simulink model "PID"  (R2023a)
settings: Solver=VariableStepAuto  StartTime=0.0  StopTime=1000  RelTol=1e-3
PreLoadFcn:
  | eta = Simulink.Signal;
  | eta.CoderInfo.StorageClass = 'ExportedGlobal';
  | eta.InitialValue = '[0 0 0 0 0 0]';
  | V = Simulink.Signal;
  | V.CoderInfo.StorageClass = 'ExportedGlobal';
  | V.InitialValue = '[0 0 0 0 0 0]';
model workspace: external: MATLAB File /home/ponbapanda/study_material/ee4901/6DOF-UUV/src/OdeRexRov.m (data not in the file)
values from neighbouring files (symbols this model uses):
  Minv = inv(M)    [OdeRexRov.m]
undefined symbols (not defined in the file or in its folder): DiscIntNeverNeededParam
libraries: slpidlib x6, simulink x1
settings Model: Creator=ponbapanda  LastModifiedBy=ponbapanda

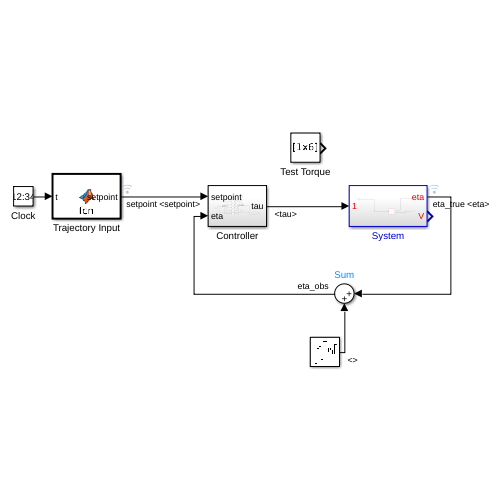
[thumbnail: Simulink's stored preview of the top-level diagram]
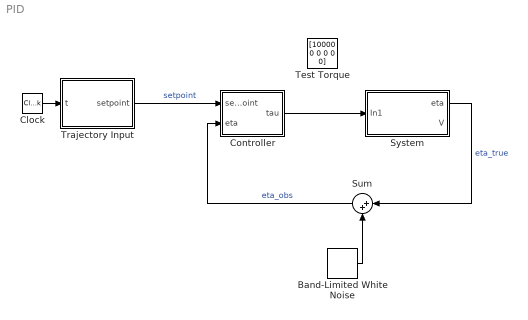
== system PID ==
  Band-Limited White Noise : simulink/Sources/Band-Limited White Noise  Cov=[0.1 0.1 0.1 0.05 0.05 0.05]  Ts=0.05  seed=[23341]
  Clock : DigitalClock  SampleTime=0.05
  Controller : Subsystem
  Sum : Sum  Inputs=|++
  System : Subsystem
  Test Torque : Constant  Value=[10000 0 0 0 0 0]
  Trajectory Input : MATLAB Function  TreatAsAtomicUnit=on
  wires:
  Clock/1 -> Trajectory Input/1(t)
  Trajectory Input/1(setpoint) -> Controller/1(setpoint)  "setpoint"
  System/1(eta) -> Sum/1  "eta_true"
  Controller/1(tau) -> System/1(In1)
  Band-Limited White Noise/1 -> Sum/2
  Sum/1 -> Controller/2(eta)  "eta_obs"

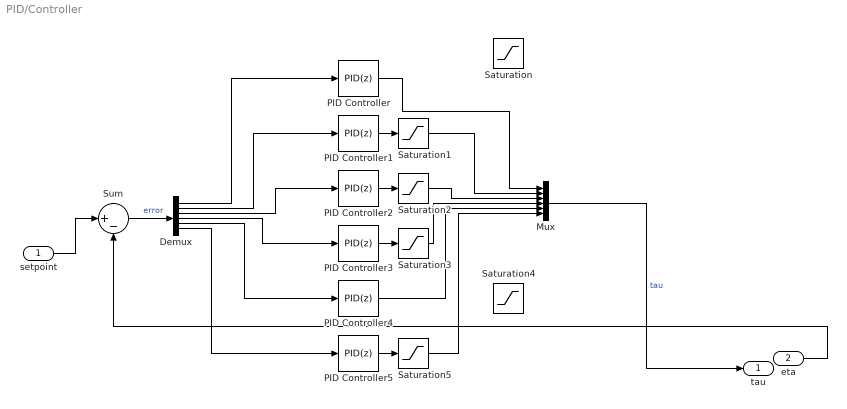
== system PID/Controller ==
  setpoint : Inport
  eta : Inport  Port=2
  Demux : Demux  Outputs=6
  Mux : Mux  Inputs=6
  PID Controller : slpidlib/PID Controller  Controller=PID  Form=Parallel  TimeDomain=Discrete-time  UseExternalTs=off  SampleTime=0.0500000000000000028  IntegratorMethod=Forward Euler  FilterMethod=Forward Euler  ControllerParametersSource=internal  P=500.000000000000000  I=10.000000000000000  UseKiTs=off  D=503.391827453152189  N=19.865241060018288  UseFilter=on  TunerSelectOption=Transfer Function Based (PID Tuner App)  InitialConditionSource=internal  InitialConditionForIntegrator=0  InitialConditionForFilter=0  DifferentiatorICPrevScaledInput=0  ExternalReset=none  TrackingMode=off  Kt=1  LimitOutput=off  SatLimitsSource=internal  UpperSaturationLimit=inf  LowerSaturationLimit=-inf  LinearizeAsGain=on  AntiWindupMode=none  Kb=1  LimitIntegrator=off  UpperIntegratorSaturationLimit=inf  LowerIntegratorSaturationLimit=-inf  POutMin=[]  POutMax=[]  IOutMin=[]  IOutMax=[]  DOutMin=[]  DOutMax=[]  NOutMin=[]  NOutMax=[]  SumOutMin=[]  SumOutMax=[]  SaturationOutMin=[]  SaturationOutMax=[]  PParamMin=[]  PParamMax=[]  IParamMin=[]  IParamMax=[]  DParamMin=[]  DParamMax=[]  NParamMin=[]  NParamMax=[]  KbParamMin=[]  KbParamMax=[]  KtParamMin=[]  KtParamMax=[]  KbOutMin=[]  KbOutMax=[]  KtOutMin=[]  KtOutMax=[]  IntegratorOutMin=[]  IntegratorOutMax=[]  FilterOutMin=[]  FilterOutMax=[]  SumI1OutMin=[]  SumI1OutMax=[]  SumI2OutMin=[]  SumI2OutMax=[]  SumI3OutMin=[]  SumI3OutMax=[]  SumI4OutMin=[]  SumI4OutMax=[]  SumDOutMin=[]  SumDOutMax=[]  DifferentiatorOutMin=[]  DifferentiatorOutMax=[]  FilterDiffOutCoefMin=[]  FilterDiffOutCoefMax=[]  ReciprocalOutMin=[]  ReciprocalOutMax=[]  SumDenOutMin=[]  SumDenOutMax=[]  SumNumOutMin=[]  SumNumOutMax=[]  DivideOutMin=[]  DivideOutMax=[]  UdiffTsProdOutMin=[]  UdiffTsProdOutMax=[]  NTsProdOutMin=[]  NTsProdOutMax=[]  UintegralTsProdOutMin=[]  UintegralTsProdOutMax=[]  UngainTsProdOutMin=[]  UngainTsProdOutMax=[]  ClampingZeroOutDataTypeStr=Inherit: Inherit via back propagation  ClampingZeroOutMin=[]  ClampingZeroOutMax=[]  FilterDenConstantOutDataTypeStr=Inherit: Inherit via back propagation  FilterDenConstantOutMin=[]  FilterDenConstantOutMax=[]  PCopyOutDataTypeStr=Inherit: Inherit via back propagation  PCopyOutMin=[]  PCopyOutMax=[]  NCopyOutDataTypeStr=Inherit: Inherit via back propagation  NCopyOutMin=[]  NCopyOutMax=[]  IntegratorContinuousStateAttributes=''  IntegratorStateMustResolveToSignalObject=off  IntegratorRTWStateStorageClass=Auto  FilterContinuousStateAttributes=''  FilterStateMustResolveToSignalObject=off  FilterRTWStateStorageClass=Auto  ParallelPVariant=InternalParameters  IdealPVariant=Disabled  IVariant=InternalParameters  DVariant=InternalParameters  IntegratorVariant=Discrete  SatVariant=Disabled  AWVariant=Passthrough  PCopyVariant=Disabled  TRVariant=Disabled  FdbkBlocksVariant=Forward  IdealPFdbkVariant=Disabled  SatFdbkVariant=Disabled  DerivativeFilterVariant=ForwardEulerFilter  NVariant=InternalParameters  NCopyVariant=Disabled  FilterICVariant=InternalICsFilter  IntegratorICVariant=InternalICs  ExternalResetVariant=Disabled  TRSumVariant=Passthrough  SumFdbkVariant=Disabled  SumVariant=Sum_PID  TsampFilterVariant=InternalTs  TsampNgainVariant=Passthrough  TsampIntegralVariant=Disabled_SignalSpec  ExternalSaturationOutDataTypeStr=Inherit: Same as second input
  PID Controller1 : slpidlib/PID Controller  Controller=PID  Form=Parallel  TimeDomain=Discrete-time  UseExternalTs=off  SampleTime=0.0500000000000000028  IntegratorMethod=Forward Euler  FilterMethod=Forward Euler  ControllerParametersSource=internal  P=500.000000000000000  I=10.000000000000000  UseKiTs=off  D=503.391827453152189  N=19.865241060018288  UseFilter=on  TunerSelectOption=Transfer Function Based (PID Tuner App)  InitialConditionSource=internal  InitialConditionForIntegrator=0  InitialConditionForFilter=0  DifferentiatorICPrevScaledInput=0  ExternalReset=none  TrackingMode=off  Kt=1  LimitOutput=off  SatLimitsSource=internal  UpperSaturationLimit=inf  LowerSaturationLimit=-inf  LinearizeAsGain=on  AntiWindupMode=none  Kb=1  LimitIntegrator=off  UpperIntegratorSaturationLimit=inf  LowerIntegratorSaturationLimit=-inf  POutMin=[]  POutMax=[]  IOutMin=[]  IOutMax=[]  DOutMin=[]  DOutMax=[]  NOutMin=[]  NOutMax=[]  SumOutMin=[]  SumOutMax=[]  SaturationOutMin=[]  SaturationOutMax=[]  PParamMin=[]  PParamMax=[]  IParamMin=[]  IParamMax=[]  DParamMin=[]  DParamMax=[]  NParamMin=[]  NParamMax=[]  KbParamMin=[]  KbParamMax=[]  KtParamMin=[]  KtParamMax=[]  KbOutMin=[]  KbOutMax=[]  KtOutMin=[]  KtOutMax=[]  IntegratorOutMin=[]  IntegratorOutMax=[]  FilterOutMin=[]  FilterOutMax=[]  SumI1OutMin=[]  SumI1OutMax=[]  SumI2OutMin=[]  SumI2OutMax=[]  SumI3OutMin=[]  SumI3OutMax=[]  SumI4OutMin=[]  SumI4OutMax=[]  SumDOutMin=[]  SumDOutMax=[]  DifferentiatorOutMin=[]  DifferentiatorOutMax=[]  FilterDiffOutCoefMin=[]  FilterDiffOutCoefMax=[]  ReciprocalOutMin=[]  ReciprocalOutMax=[]  SumDenOutMin=[]  SumDenOutMax=[]  SumNumOutMin=[]  SumNumOutMax=[]  DivideOutMin=[]  DivideOutMax=[]  UdiffTsProdOutMin=[]  UdiffTsProdOutMax=[]  NTsProdOutMin=[]  NTsProdOutMax=[]  UintegralTsProdOutMin=[]  UintegralTsProdOutMax=[]  UngainTsProdOutMin=[]  UngainTsProdOutMax=[]  ClampingZeroOutDataTypeStr=Inherit: Inherit via back propagation  ClampingZeroOutMin=[]  ClampingZeroOutMax=[]  FilterDenConstantOutDataTypeStr=Inherit: Inherit via back propagation  FilterDenConstantOutMin=[]  FilterDenConstantOutMax=[]  PCopyOutDataTypeStr=Inherit: Inherit via back propagation  PCopyOutMin=[]  PCopyOutMax=[]  NCopyOutDataTypeStr=Inherit: Inherit via back propagation  NCopyOutMin=[]  NCopyOutMax=[]  IntegratorContinuousStateAttributes=''  IntegratorStateMustResolveToSignalObject=off  IntegratorRTWStateStorageClass=Auto  FilterContinuousStateAttributes=''  FilterStateMustResolveToSignalObject=off  FilterRTWStateStorageClass=Auto  ParallelPVariant=InternalParameters  IdealPVariant=Disabled  IVariant=InternalParameters  DVariant=InternalParameters  IntegratorVariant=Discrete  SatVariant=Disabled  AWVariant=Passthrough  PCopyVariant=Disabled  TRVariant=Disabled  FdbkBlocksVariant=Forward  IdealPFdbkVariant=Disabled  SatFdbkVariant=Disabled  DerivativeFilterVariant=ForwardEulerFilter  NVariant=InternalParameters  NCopyVariant=Disabled  FilterICVariant=InternalICsFilter  IntegratorICVariant=InternalICs  ExternalResetVariant=Disabled  TRSumVariant=Passthrough  SumFdbkVariant=Disabled  SumVariant=Sum_PID  TsampFilterVariant=InternalTs  TsampNgainVariant=Passthrough  TsampIntegralVariant=Disabled_SignalSpec  ExternalSaturationOutDataTypeStr=Inherit: Same as second input
  PID Controller2 : slpidlib/PID Controller  Controller=PID  Form=Parallel  TimeDomain=Discrete-time  UseExternalTs=off  SampleTime=0.0500000000000000028  IntegratorMethod=Forward Euler  FilterMethod=Forward Euler  ControllerParametersSource=internal  P=500.000000000000000  I=0.000000000000000  UseKiTs=off  D=503.391827453152189  N=19.865241060018288  UseFilter=on  TunerSelectOption=Transfer Function Based (PID Tuner App)  InitialConditionSource=internal  InitialConditionForIntegrator=0  InitialConditionForFilter=0  DifferentiatorICPrevScaledInput=0  ExternalReset=none  TrackingMode=off  Kt=1  LimitOutput=off  SatLimitsSource=internal  UpperSaturationLimit=inf  LowerSaturationLimit=-inf  LinearizeAsGain=on  AntiWindupMode=none  Kb=1  LimitIntegrator=off  UpperIntegratorSaturationLimit=inf  LowerIntegratorSaturationLimit=-inf  POutMin=[]  POutMax=[]  IOutMin=[]  IOutMax=[]  DOutMin=[]  DOutMax=[]  NOutMin=[]  NOutMax=[]  SumOutMin=[]  SumOutMax=[]  SaturationOutMin=[]  SaturationOutMax=[]  PParamMin=[]  PParamMax=[]  IParamMin=[]  IParamMax=[]  DParamMin=[]  DParamMax=[]  NParamMin=[]  NParamMax=[]  KbParamMin=[]  KbParamMax=[]  KtParamMin=[]  KtParamMax=[]  KbOutMin=[]  KbOutMax=[]  KtOutMin=[]  KtOutMax=[]  IntegratorOutMin=[]  IntegratorOutMax=[]  FilterOutMin=[]  FilterOutMax=[]  SumI1OutMin=[]  SumI1OutMax=[]  SumI2OutMin=[]  SumI2OutMax=[]  SumI3OutMin=[]  SumI3OutMax=[]  SumI4OutMin=[]  SumI4OutMax=[]  SumDOutMin=[]  SumDOutMax=[]  DifferentiatorOutMin=[]  DifferentiatorOutMax=[]  FilterDiffOutCoefMin=[]  FilterDiffOutCoefMax=[]  ReciprocalOutMin=[]  ReciprocalOutMax=[]  SumDenOutMin=[]  SumDenOutMax=[]  SumNumOutMin=[]  SumNumOutMax=[]  DivideOutMin=[]  DivideOutMax=[]  UdiffTsProdOutMin=[]  UdiffTsProdOutMax=[]  NTsProdOutMin=[]  NTsProdOutMax=[]  UintegralTsProdOutMin=[]  UintegralTsProdOutMax=[]  UngainTsProdOutMin=[]  UngainTsProdOutMax=[]  ClampingZeroOutDataTypeStr=Inherit: Inherit via back propagation  ClampingZeroOutMin=[]  ClampingZeroOutMax=[]  FilterDenConstantOutDataTypeStr=Inherit: Inherit via back propagation  FilterDenConstantOutMin=[]  FilterDenConstantOutMax=[]  PCopyOutDataTypeStr=Inherit: Inherit via back propagation  PCopyOutMin=[]  PCopyOutMax=[]  NCopyOutDataTypeStr=Inherit: Inherit via back propagation  NCopyOutMin=[]  NCopyOutMax=[]  IntegratorContinuousStateAttributes=''  IntegratorStateMustResolveToSignalObject=off  IntegratorRTWStateStorageClass=Auto  FilterContinuousStateAttributes=''  FilterStateMustResolveToSignalObject=off  FilterRTWStateStorageClass=Auto  ParallelPVariant=InternalParameters  IdealPVariant=Disabled  IVariant=InternalParameters  DVariant=InternalParameters  IntegratorVariant=Discrete  SatVariant=Disabled  AWVariant=Passthrough  PCopyVariant=Disabled  TRVariant=Disabled  FdbkBlocksVariant=Forward  IdealPFdbkVariant=Disabled  SatFdbkVariant=Disabled  DerivativeFilterVariant=ForwardEulerFilter  NVariant=InternalParameters  NCopyVariant=Disabled  FilterICVariant=InternalICsFilter  IntegratorICVariant=InternalICs  ExternalResetVariant=Disabled  TRSumVariant=Passthrough  SumFdbkVariant=Disabled  SumVariant=Sum_PID  TsampFilterVariant=InternalTs  TsampNgainVariant=Passthrough  TsampIntegralVariant=Disabled_SignalSpec  ExternalSaturationOutDataTypeStr=Inherit: Same as second input
  PID Controller3 : slpidlib/PID Controller  Controller=PID  Form=Parallel  TimeDomain=Discrete-time  UseExternalTs=off  SampleTime=0.0500000000000000028  IntegratorMethod=Forward Euler  FilterMethod=Forward Euler  ControllerParametersSource=internal  P=5000.000000000000000  I=500.000000000000000  UseKiTs=off  D=503.391827453152189  N=19.865241060018288  UseFilter=on  TunerSelectOption=Transfer Function Based (PID Tuner App)  InitialConditionSource=internal  InitialConditionForIntegrator=0  InitialConditionForFilter=0  DifferentiatorICPrevScaledInput=0  ExternalReset=none  TrackingMode=off  Kt=1  LimitOutput=off  SatLimitsSource=internal  UpperSaturationLimit=inf  LowerSaturationLimit=-inf  LinearizeAsGain=on  AntiWindupMode=none  Kb=1  LimitIntegrator=off  UpperIntegratorSaturationLimit=inf  LowerIntegratorSaturationLimit=-inf  POutMin=[]  POutMax=[]  IOutMin=[]  IOutMax=[]  DOutMin=[]  DOutMax=[]  NOutMin=[]  NOutMax=[]  SumOutMin=[]  SumOutMax=[]  SaturationOutMin=[]  SaturationOutMax=[]  PParamMin=[]  PParamMax=[]  IParamMin=[]  IParamMax=[]  DParamMin=[]  DParamMax=[]  NParamMin=[]  NParamMax=[]  KbParamMin=[]  KbParamMax=[]  KtParamMin=[]  KtParamMax=[]  KbOutMin=[]  KbOutMax=[]  KtOutMin=[]  KtOutMax=[]  IntegratorOutMin=[]  IntegratorOutMax=[]  FilterOutMin=[]  FilterOutMax=[]  SumI1OutMin=[]  SumI1OutMax=[]  SumI2OutMin=[]  SumI2OutMax=[]  SumI3OutMin=[]  SumI3OutMax=[]  SumI4OutMin=[]  SumI4OutMax=[]  SumDOutMin=[]  SumDOutMax=[]  DifferentiatorOutMin=[]  DifferentiatorOutMax=[]  FilterDiffOutCoefMin=[]  FilterDiffOutCoefMax=[]  ReciprocalOutMin=[]  ReciprocalOutMax=[]  SumDenOutMin=[]  SumDenOutMax=[]  SumNumOutMin=[]  SumNumOutMax=[]  DivideOutMin=[]  DivideOutMax=[]  UdiffTsProdOutMin=[]  UdiffTsProdOutMax=[]  NTsProdOutMin=[]  NTsProdOutMax=[]  UintegralTsProdOutMin=[]  UintegralTsProdOutMax=[]  UngainTsProdOutMin=[]  UngainTsProdOutMax=[]  ClampingZeroOutDataTypeStr=Inherit: Inherit via back propagation  ClampingZeroOutMin=[]  ClampingZeroOutMax=[]  FilterDenConstantOutDataTypeStr=Inherit: Inherit via back propagation  FilterDenConstantOutMin=[]  FilterDenConstantOutMax=[]  PCopyOutDataTypeStr=Inherit: Inherit via back propagation  PCopyOutMin=[]  PCopyOutMax=[]  NCopyOutDataTypeStr=Inherit: Inherit via back propagation  NCopyOutMin=[]  NCopyOutMax=[]  IntegratorContinuousStateAttributes=''  IntegratorStateMustResolveToSignalObject=off  IntegratorRTWStateStorageClass=Auto  FilterContinuousStateAttributes=''  FilterStateMustResolveToSignalObject=off  FilterRTWStateStorageClass=Auto  ParallelPVariant=InternalParameters  IdealPVariant=Disabled  IVariant=InternalParameters  DVariant=InternalParameters  IntegratorVariant=Discrete  SatVariant=Disabled  AWVariant=Passthrough  PCopyVariant=Disabled  TRVariant=Disabled  FdbkBlocksVariant=Forward  IdealPFdbkVariant=Disabled  SatFdbkVariant=Disabled  DerivativeFilterVariant=ForwardEulerFilter  NVariant=InternalParameters  NCopyVariant=Disabled  FilterICVariant=InternalICsFilter  IntegratorICVariant=InternalICs  ExternalResetVariant=Disabled  TRSumVariant=Passthrough  SumFdbkVariant=Disabled  SumVariant=Sum_PID  TsampFilterVariant=InternalTs  TsampNgainVariant=Passthrough  TsampIntegralVariant=Disabled_SignalSpec  ExternalSaturationOutDataTypeStr=Inherit: Same as second input
  PID Controller4 : slpidlib/PID Controller  Controller=PID  Form=Parallel  TimeDomain=Discrete-time  UseExternalTs=off  SampleTime=0.0500000000000000028  IntegratorMethod=Forward Euler  FilterMethod=Forward Euler  ControllerParametersSource=internal  P=5000.000000000000000  I=500.000000000000000  UseKiTs=off  D=503.391827453152189  N=19.865241060018288  UseFilter=on  TunerSelectOption=Transfer Function Based (PID Tuner App)  InitialConditionSource=internal  InitialConditionForIntegrator=0  InitialConditionForFilter=0  DifferentiatorICPrevScaledInput=0  ExternalReset=none  TrackingMode=off  Kt=1  LimitOutput=off  SatLimitsSource=internal  UpperSaturationLimit=inf  LowerSaturationLimit=-inf  LinearizeAsGain=on  AntiWindupMode=none  Kb=1  LimitIntegrator=off  UpperIntegratorSaturationLimit=inf  LowerIntegratorSaturationLimit=-inf  POutMin=[]  POutMax=[]  IOutMin=[]  IOutMax=[]  DOutMin=[]  DOutMax=[]  NOutMin=[]  NOutMax=[]  SumOutMin=[]  SumOutMax=[]  SaturationOutMin=[]  SaturationOutMax=[]  PParamMin=[]  PParamMax=[]  IParamMin=[]  IParamMax=[]  DParamMin=[]  DParamMax=[]  NParamMin=[]  NParamMax=[]  KbParamMin=[]  KbParamMax=[]  KtParamMin=[]  KtParamMax=[]  KbOutMin=[]  KbOutMax=[]  KtOutMin=[]  KtOutMax=[]  IntegratorOutMin=[]  IntegratorOutMax=[]  FilterOutMin=[]  FilterOutMax=[]  SumI1OutMin=[]  SumI1OutMax=[]  SumI2OutMin=[]  SumI2OutMax=[]  SumI3OutMin=[]  SumI3OutMax=[]  SumI4OutMin=[]  SumI4OutMax=[]  SumDOutMin=[]  SumDOutMax=[]  DifferentiatorOutMin=[]  DifferentiatorOutMax=[]  FilterDiffOutCoefMin=[]  FilterDiffOutCoefMax=[]  ReciprocalOutMin=[]  ReciprocalOutMax=[]  SumDenOutMin=[]  SumDenOutMax=[]  SumNumOutMin=[]  SumNumOutMax=[]  DivideOutMin=[]  DivideOutMax=[]  UdiffTsProdOutMin=[]  UdiffTsProdOutMax=[]  NTsProdOutMin=[]  NTsProdOutMax=[]  UintegralTsProdOutMin=[]  UintegralTsProdOutMax=[]  UngainTsProdOutMin=[]  UngainTsProdOutMax=[]  ClampingZeroOutDataTypeStr=Inherit: Inherit via back propagation  ClampingZeroOutMin=[]  ClampingZeroOutMax=[]  FilterDenConstantOutDataTypeStr=Inherit: Inherit via back propagation  FilterDenConstantOutMin=[]  FilterDenConstantOutMax=[]  PCopyOutDataTypeStr=Inherit: Inherit via back propagation  PCopyOutMin=[]  PCopyOutMax=[]  NCopyOutDataTypeStr=Inherit: Inherit via back propagation  NCopyOutMin=[]  NCopyOutMax=[]  IntegratorContinuousStateAttributes=''  IntegratorStateMustResolveToSignalObject=off  IntegratorRTWStateStorageClass=Auto  FilterContinuousStateAttributes=''  FilterStateMustResolveToSignalObject=off  FilterRTWStateStorageClass=Auto  ParallelPVariant=InternalParameters  IdealPVariant=Disabled  IVariant=InternalParameters  DVariant=InternalParameters  IntegratorVariant=Discrete  SatVariant=Disabled  AWVariant=Passthrough  PCopyVariant=Disabled  TRVariant=Disabled  FdbkBlocksVariant=Forward  IdealPFdbkVariant=Disabled  SatFdbkVariant=Disabled  DerivativeFilterVariant=ForwardEulerFilter  NVariant=InternalParameters  NCopyVariant=Disabled  FilterICVariant=InternalICsFilter  IntegratorICVariant=InternalICs  ExternalResetVariant=Disabled  TRSumVariant=Passthrough  SumFdbkVariant=Disabled  SumVariant=Sum_PID  TsampFilterVariant=InternalTs  TsampNgainVariant=Passthrough  TsampIntegralVariant=Disabled_SignalSpec  ExternalSaturationOutDataTypeStr=Inherit: Same as second input
  PID Controller5 : slpidlib/PID Controller  Controller=PID  Form=Parallel  TimeDomain=Discrete-time  UseExternalTs=off  SampleTime=0.0500000000000000028  IntegratorMethod=Forward Euler  FilterMethod=Forward Euler  ControllerParametersSource=internal  P=5000.000000000000000  I=500.000000000000000  UseKiTs=off  D=503.391827453152189  N=19.865241060018288  UseFilter=on  TunerSelectOption=Transfer Function Based (PID Tuner App)  InitialConditionSource=internal  InitialConditionForIntegrator=0  InitialConditionForFilter=0  DifferentiatorICPrevScaledInput=0  ExternalReset=none  TrackingMode=off  Kt=1  LimitOutput=off  SatLimitsSource=internal  UpperSaturationLimit=inf  LowerSaturationLimit=-inf  LinearizeAsGain=on  AntiWindupMode=none  Kb=1  LimitIntegrator=off  UpperIntegratorSaturationLimit=inf  LowerIntegratorSaturationLimit=-inf  POutMin=[]  POutMax=[]  IOutMin=[]  IOutMax=[]  DOutMin=[]  DOutMax=[]  NOutMin=[]  NOutMax=[]  SumOutMin=[]  SumOutMax=[]  SaturationOutMin=[]  SaturationOutMax=[]  PParamMin=[]  PParamMax=[]  IParamMin=[]  IParamMax=[]  DParamMin=[]  DParamMax=[]  NParamMin=[]  NParamMax=[]  KbParamMin=[]  KbParamMax=[]  KtParamMin=[]  KtParamMax=[]  KbOutMin=[]  KbOutMax=[]  KtOutMin=[]  KtOutMax=[]  IntegratorOutMin=[]  IntegratorOutMax=[]  FilterOutMin=[]  FilterOutMax=[]  SumI1OutMin=[]  SumI1OutMax=[]  SumI2OutMin=[]  SumI2OutMax=[]  SumI3OutMin=[]  SumI3OutMax=[]  SumI4OutMin=[]  SumI4OutMax=[]  SumDOutMin=[]  SumDOutMax=[]  DifferentiatorOutMin=[]  DifferentiatorOutMax=[]  FilterDiffOutCoefMin=[]  FilterDiffOutCoefMax=[]  ReciprocalOutMin=[]  ReciprocalOutMax=[]  SumDenOutMin=[]  SumDenOutMax=[]  SumNumOutMin=[]  SumNumOutMax=[]  DivideOutMin=[]  DivideOutMax=[]  UdiffTsProdOutMin=[]  UdiffTsProdOutMax=[]  NTsProdOutMin=[]  NTsProdOutMax=[]  UintegralTsProdOutMin=[]  UintegralTsProdOutMax=[]  UngainTsProdOutMin=[]  UngainTsProdOutMax=[]  ClampingZeroOutDataTypeStr=Inherit: Inherit via back propagation  ClampingZeroOutMin=[]  ClampingZeroOutMax=[]  FilterDenConstantOutDataTypeStr=Inherit: Inherit via back propagation  FilterDenConstantOutMin=[]  FilterDenConstantOutMax=[]  PCopyOutDataTypeStr=Inherit: Inherit via back propagation  PCopyOutMin=[]  PCopyOutMax=[]  NCopyOutDataTypeStr=Inherit: Inherit via back propagation  NCopyOutMin=[]  NCopyOutMax=[]  IntegratorContinuousStateAttributes=''  IntegratorStateMustResolveToSignalObject=off  IntegratorRTWStateStorageClass=Auto  FilterContinuousStateAttributes=''  FilterStateMustResolveToSignalObject=off  FilterRTWStateStorageClass=Auto  ParallelPVariant=InternalParameters  IdealPVariant=Disabled  IVariant=InternalParameters  DVariant=InternalParameters  IntegratorVariant=Discrete  SatVariant=Disabled  AWVariant=Passthrough  PCopyVariant=Disabled  TRVariant=Disabled  FdbkBlocksVariant=Forward  IdealPFdbkVariant=Disabled  SatFdbkVariant=Disabled  DerivativeFilterVariant=ForwardEulerFilter  NVariant=InternalParameters  NCopyVariant=Disabled  FilterICVariant=InternalICsFilter  IntegratorICVariant=InternalICs  ExternalResetVariant=Disabled  TRSumVariant=Passthrough  SumFdbkVariant=Disabled  SumVariant=Sum_PID  TsampFilterVariant=InternalTs  TsampNgainVariant=Passthrough  TsampIntegralVariant=Disabled_SignalSpec  ExternalSaturationOutDataTypeStr=Inherit: Same as second input
  Saturation : Saturate  UpperLimit=8000  LowerLimit=-8000  LinearizeAsGain=off  ZeroCross=off
  Saturation1 : Saturate  UpperLimit=8000  LowerLimit=-8000  LinearizeAsGain=off  ZeroCross=off
  Saturation2 : Saturate  UpperLimit=8000  LowerLimit=-8000  LinearizeAsGain=off  ZeroCross=off
  Saturation3 : Saturate  UpperLimit=100000  LowerLimit=-100000  LinearizeAsGain=off  ZeroCross=off
  Saturation4 : Saturate  UpperLimit=100000  LowerLimit=-100000  LinearizeAsGain=off  ZeroCross=off
  Saturation5 : Saturate  UpperLimit=100000  LowerLimit=-100000  LinearizeAsGain=off  ZeroCross=off
  Sum : Sum  Inputs=|+-
  tau : Outport
  wires:
  PID Controller5/1 -> Saturation5/1
  setpoint/1 -> Sum/1
  PID Controller1/1 -> Saturation1/1
  Mux/1 -> tau/1  "tau"
  PID Controller4/1 -> Mux/5
  PID Controller/1 -> Mux/1
  Demux/5 -> PID Controller4/1
  eta/1 -> Sum/2
  PID Controller3/1 -> Saturation3/1
  Demux/2 -> PID Controller1/1
  Demux/4 -> PID Controller3/1
  Saturation2/1 -> Mux/3
  Demux/3 -> PID Controller2/1
  Demux/6 -> PID Controller5/1
  Saturation5/1 -> Mux/6
  Saturation3/1 -> Mux/4
  PID Controller2/1 -> Saturation2/1
  Sum/1 -> Demux/1  "error"
  Saturation1/1 -> Mux/2
  Demux/1 -> PID Controller/1

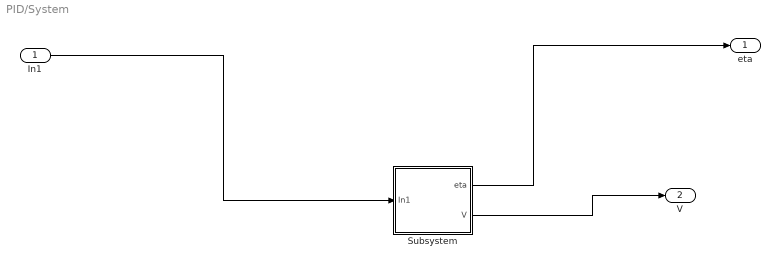
== system PID/System ==
  In1 : Inport
  Subsystem : Subsystem
  eta : Outport
  V : Outport  Port=2
  wires:
  In1/1 -> Subsystem/1(In1)
  Subsystem/1(eta) -> eta/1
  Subsystem/2(V) -> V/1

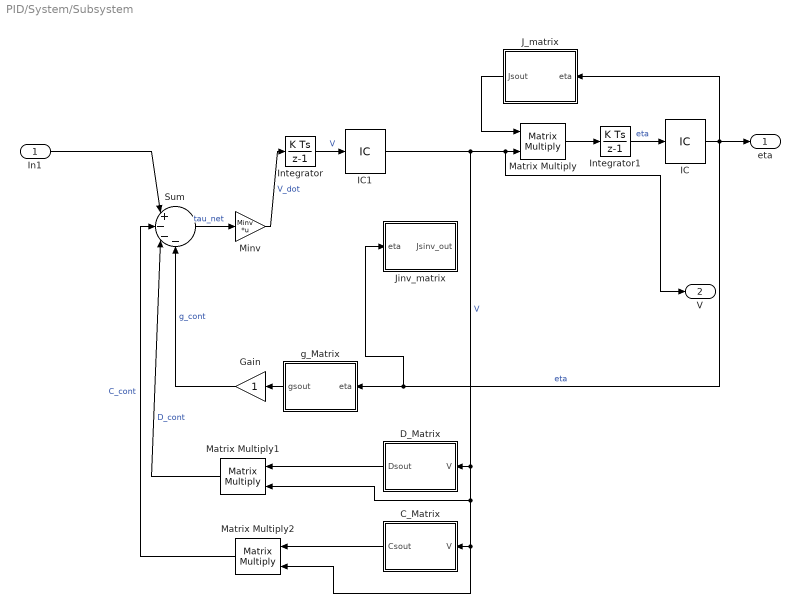
== system PID/System/Subsystem ==
  In1 : Inport
  C_Matrix : MATLAB Function  TreatAsAtomicUnit=on
  D_Matrix : MATLAB Function  TreatAsAtomicUnit=on
  Gain : Gain
  IC : InitialCondition  Value=[0 0 0 0 0 0]
  IC1 : InitialCondition  Value=[0 0 0 0 0 0]
  Integrator : DiscreteIntegrator  SampleTime=0.05  ICPrevOutput=DiscIntNeverNeededParam  ICPrevScaledInput=DiscIntNeverNeededParam  mask(DiscretizedDiscreteIntegrator){}
      mask init:
      | %zoh
  Integrator1 : DiscreteIntegrator  SampleTime=0.05  ICPrevOutput=DiscIntNeverNeededParam  ICPrevScaledInput=DiscIntNeverNeededParam  mask(DiscretizedDiscreteIntegrator){}
      mask init:
      | %zoh
  J_matrix : MATLAB Function  TreatAsAtomicUnit=on
  Jinv_matrix : MATLAB Function  TreatAsAtomicUnit=on
  Matrix Multiply : Product  Multiplication=Matrix(*)
  Matrix Multiply1 : Product  Multiplication=Matrix(*)
  Matrix Multiply2 : Product  Multiplication=Matrix(*)
  Minv : Gain  Gain=Minv  Multiplication=Matrix(K*u) (u vector)
  Sum : Sum  Inputs=|+---
  g_Matrix : MATLAB Function  TreatAsAtomicUnit=on
  eta : Outport
  V : Outport  Port=2
  wires:
  J_matrix/1(Jsout) -> Matrix Multiply/1
  Matrix Multiply1/1 -> Sum/3  "D_cont"
  Matrix Multiply2/1 -> Sum/2  "C_cont"
  D_Matrix/1(Dsout) -> Matrix Multiply1/1
  C_Matrix/1(Csout) -> Matrix Multiply2/1
  Matrix Multiply/1 -> Integrator1/1
  Gain/1 -> Sum/4  "g_cont"
  IC1/1 -> Matrix Multiply1/2, Matrix Multiply2/2, C_Matrix/1(V), D_Matrix/1(V), V/1, Matrix Multiply/2  "V"
  Minv/1 -> Integrator/1  "V_dot"
  In1/1 -> Sum/1
  Integrator1/1 -> IC/1  "eta"
  IC/1 -> J_matrix/1(eta), Jinv_matrix/1(eta), g_Matrix/1(eta), eta/1  "eta"
  Integrator/1 -> IC1/1  "V"
  Sum/1 -> Minv/1  "tau_net"
  g_Matrix/1(gsout) -> Gain/1

== matlab function PID/System/Subsystem/J_matrix ==
  data: eta input; Jsout output
function Jsout = Js(eta)
x = eta(1,:);
y = eta(2,:);
z = eta(3,:);
phi = eta(4,:);
theta = eta(5,:);
psi = eta(6,:);
t2 = cos(phi);
t3 = cos(psi);
t4 = cos(theta);
t5 = sin(phi);
t6 = sin(psi);
t7 = sin(theta);
t8 = tan(theta);
t9 = 1.0./t4;
Jsout = reshape([t3.*t4,t4.*t6,t7.*-1.0,0.0,0.0,0.0,t2.*t6.*-1.0+t3.*t5.*t7,t2.*t3+t5.*t6.*t7,t4.*t5,0.0,0.0,0.0,t5.*t6+t2.*t3.*t7,t3.*t5.*-1.0+t2.*t6.*t7,t2.*t4,0.0,0.0,0.0,0.0,0.0,0.0,1.0,0.0,0.0,0.0,0.0,0.0,t5.*t8,t2,t5.*t9,0.0,0.0,0.0,t2.*t8,t5.*-1.0,t2.*t9],[6,6]);
end

== matlab function PID/System/Subsystem/D_Matrix ==
  data: V input; Dsout output
function Dsout = Ds(V)
u = V(1,:);
v = V(2,:);
w = V(3,:);
p = V(4,:);
q = V(5,:);
r = V(6,:);
Dsout = reshape([abs(u).*7.4822e+2+7.482e+1,0.0,0.0,0.0,0.0,0.0,0.0,abs(v).*9.9253e+2+6.948e+1,0.0,0.0,0.0,0.0,0.0,0.0,abs(w).*1.82101e+3+7.284e+2,0.0,0.0,0.0,0.0,0.0,0.0,abs(p).*6.72e+2+2.688e+2,0.0,0.0,0.0,0.0,0.0,0.0,abs(q).*7.7444e+2+3.0977e+2,0.0,0.0,0.0,0.0,0.0,0.0,abs(r).*5.2327e+2+1.05e+2],[6,6]);

== matlab function PID/System/Subsystem/C_Matrix ==
  data: V input; Csout output
function Csout = Cs(V)

u = V(1,:);
v = V(2,:);
w = V(3,:);
p = V(4,:);
q = V(5,:);
r = V(6,:);
t2 = p.*1.06029e+3;
t3 = p.*-8.5426;
t4 = p.*8.5426;
t5 = p.*8.587;
t6 = q.*8.587;
t7 = u.*8.5426;
t8 = v.*-1.222e+3;
t9 = v.*1.222e+3;
t10 = q.*-1.6554e+2;
t11 = q.*1.6554e+2;
t12 = u.*1.6554e+2;
t13 = r.*-1.0774e+1;
t14 = r.*1.0774e+1;
t15 = w.*1.0775e+1;
t16 = q.*-5.8488;
t17 = q.*5.8488;
t18 = q.*1.4838;
t19 = r.*1.4838;
t20 = q.*-3.8642e+2;
t21 = q.*3.8642e+2;
t22 = p.*-6.1112;
t23 = p.*6.1112;
t24 = v.*5.8488;
t25 = p.*-4.0944e+2;
t26 = p.*4.0944e+2;
t27 = u.*-7.7979e+2;
t28 = u.*7.7979e+2;
t29 = q.*1.63689e+3;
t30 = w.*3.8642e+2;
t31 = w.*6.1112;
t32 = u.*-1.0332e+2;
t33 = u.*1.0332e+2;
t34 = v.*4.0944e+2;
t35 = v.*-5.129e+1;
t36 = v.*5.129e+1;
t37 = p.*5.4429e+1;
t38 = w.*-5.129e+1;
t39 = w.*5.129e+1;
t40 = w.*-1.0332e+2;
t41 = w.*1.0332e+2;
t42 = r.*5.4429e+1;
t43 = u.*-6.8773;
t44 = u.*6.8773;
t45 = v.*-6.8773;
t46 = v.*6.8773;
t47 = p.*1.86287e+3;
t48 = r.*9.1555e+2;
t49 = q.*1.86287e+3;
t50 = r.*1.86287e+3;
t51 = w.*-3.6599e+3;
t52 = w.*3.6599e+3;
t53 = r.*-7.8033;
t54 = r.*7.8033;
t55 = r.*-6.2726e+1;
t56 = r.*6.2726e+1;
t57 = u.*7.8033;
t58 = v.*6.2726e+1;
t59 = t3+t11+t27+t41+t46+t54;
t60 = t4+t10+t28+t40+t45+t53;
t61 = t13+t21+t22+t33+t35+t51;
t62 = t14+t20+t23+t32+t36+t52;
t63 = t8+t17+t25+t38+t44+t55;
t64 = t9+t16+t26+t39+t43+t56;
Csout = reshape([0.0,t50,-t49,0.0,t61,t64,-t50,0.0,t47,t62,0.0,t59,t49,-t47,0.0,t63,t60,0.0,0.0,t61,t64,0.0,-t15-t18-t37-t48+t57-t58,-t5-t12+t19-t24+t29-t30,t62,0.0,t59,t15+t18+t37+t48-t57+t58,0.0,-t2+t6-t7-t31-t34-t42,t63,t60,0.0,t5+t12-t19+t24-t29+t30,t2-t6+t7+t31+t34+t42,0.0],[6,6]);
end

== matlab function PID/System/Subsystem/Jinv_matrix ==
  data: eta input; Jsinv_out output
function Jsinv_out = Jsinv(eta)

x = eta(1,:);
y = eta(2,:);
z = eta(3,:);
phi = eta(4,:);
theta = eta(5,:);
psi = eta(6,:);
t2 = cos(phi);
t3 = cos(psi);
t4 = cos(theta);
t5 = sin(phi);
t6 = sin(psi);
t7 = sin(theta);
t8 = t2.^2;
t9 = t3.^2;
t10 = t4.^2;
t11 = t5.^2;
t12 = t6.^2;
t13 = t7.^2;
t14 = t8.*t10;
t15 = t9.*t10;
t16 = t8+t11;
t17 = t8.*t13;
t18 = t10.*t11;
t19 = t9.*t13;
t20 = t10.*t12;
t21 = t11.*t13;
t22 = t12.*t13;
t23 = 1.0./t16;
t24 = t9.*t17;
t25 = t12.*t14;
t26 = t11.*t15;
t27 = t12.*t17;
t28 = t11.*t19;
t29 = t12.*t18;
t30 = t12.*t21;
t31 = t9.*t14;
t32 = t14+t17+t18+t21;
t33 = t15+t19+t20+t22;
t34 = 1.0./t32;
t35 = 1.0./t33;
t36 = t24+t25+t26+t27+t28+t29+t30+t31;
t37 = 1.0./t36;
Jsinv_out = reshape([t3.*t4.*t35.*1.0,t37.*(t3.*t5.*t7.*-1.0+t2.*t6.*t10+t2.*t6.*t13).*-1.0,t37.*(t2.*t3.*t7+t5.*t6.*t10+t5.*t6.*t13).*1.0,0.0,0.0,0.0,t4.*t6.*t35.*1.0,t37.*(t2.*t3.*t10+t2.*t3.*t13+t5.*t6.*t7).*1.0,t37.*(-t2.*t6.*t7+t3.*t5.*t10.*1.0+t3.*t5.*t13.*1.0).*-1.0,0.0,0.0,0.0,(t7.*-1.0)./(t10+t13),t4.*t5.*t34.*1.0,t2.*t4.*t34.*1.0,0.0,0.0,0.0,0.0,0.0,0.0,1.0,0.0,0.0,0.0,0.0,0.0,0.0,t2.*t23.*1.0,t5.*t23.*-1.0,0.0,0.0,0.0,t4.*tan(theta).*-1.0,t4.*t5.*t23.*1.0,t2.*t4.*t23.*1.0],[6,6]);
end

== matlab function PID/Trajectory Input ==
  data: t input; setpoint output
function setpoint = fcn(t)
%if t>400
%    setpoint = [0.05*(t-400);0;0;0;0;0];
%elseif t>200
%    setpoint = [0.05*(400-t);0;0;0;0;0];
%else
%    setpoint = [0.05*t;0;0;0;0;0];
%setpoint = [0.5*sin(t/10);0;0;0;0;0];
%setpoint = [0;0.5*sin(t/10);0;0;0;0];
%setpoint = [0.5*cos(t/10);0;0.5*sin(t/10);0;0;0];
%setpoint = [0;0;0;1.5*sin(t/10);0;0];
%setpoint = [0;0;0;0;0;0.5*sin(t/10)];
setpoint = [3*t;0;0;0;0.52*sin(t);0];
end

== matlab function PID/System/Subsystem/g_Matrix ==
  data: eta input; gsout output
function gsout = gs(eta)
x = eta(1,:);
y = eta(2,:);
z = eta(3,:);
phi = eta(4,:);
theta = eta(5,:);
psi = eta(6,:);
t2 = cos(phi);
t3 = cos(theta);
t4 = sin(phi);
t5 = sin(theta);
gsout = [t5.*-2.094180000000051e+2;t3.*t4.*2.094180000000051e+2;t2.*t3.*2.094180000000051e+2;t2.*t3.*-1.423280935999937e+2+t3.*t4.*7.157069849600084e+3;t5.*7.157069849600084e+3-t2.*t3.*1.51939860960003e+3;t5.*-1.423280935999937e+2+t3.*t4.*1.51939860960003e+3];
end
